simulink model "track_generator"  (R2022b)
settings: Solver=VariableStepAuto  StartTime=0.0  StopTime=120  RelTol=1e-3
values from neighbouring files (symbols this model uses):
  v_ref = 5    [trajectory_test.m]
  wp = wpt(L,vx_ref)    [trajectory_test_2.m]    (also in vehicle_lateral_control_LMIs_3states.m = wpt(L,vx_track); vehicle_lateral_control_LMIs_3states_auto.m = wpt(L,vx_track))
settings Model: Creator=phatdo  LastModifiedBy=phatdo
settings DataIOCC: ReturnWorkspaceOutputs=off

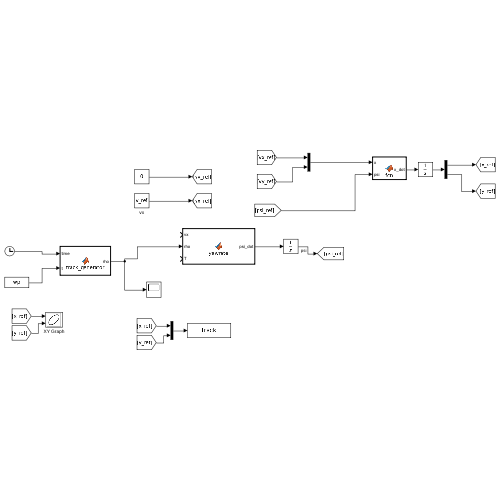
[thumbnail: Simulink's stored preview of the top-level diagram]
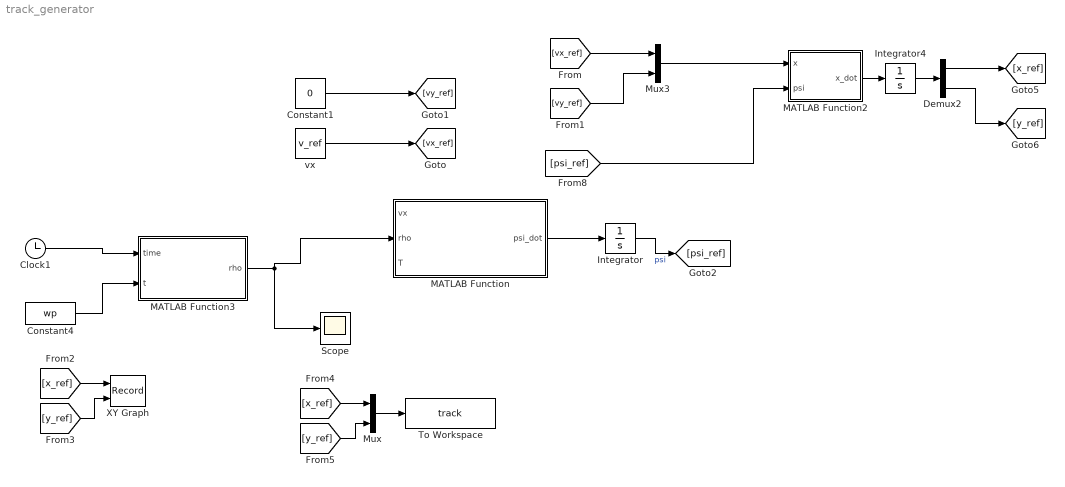
== system track_generator ==
  Clock1 : Clock
  Constant1 : Constant  Value=0
  Constant4 : Constant  Value=wp
  Demux2 : Demux  Outputs=2
  Integrator : Integrator
  Integrator4 : Integrator
  MATLAB Function : MATLAB Function  TreatAsAtomicUnit=on
  MATLAB Function2 : MATLAB Function  TreatAsAtomicUnit=on
  MATLAB Function3 : MATLAB Function  TreatAsAtomicUnit=on
  Mux : Mux  Inputs=2
  Mux3 : Mux  Inputs=2
  Scope : Scope
  To Workspace : ToWorkspace  VariableName=track  SaveFormat=Timeseries  SampleTime=-1
  XY Graph : Record  FileSettingsInternal="{\"entries\":[{\"content\":{\"excelSettings\":{\"content\":{},\"type\":\"Streamout.ExcelSettings\"}},\"type\":\"Streamout.FileSettingStorage\",\"uuid\":\"d2604bc3-c04d-4145-9e1e-7ef3e8a79466\"}],\"packageUris\":[\"http://schema.mathworks.com/mf0/streamout_blocks/R2020a\"],\"version\":\"1.0\"}"  Layout=[1 1]  SignalsInternal="{\"entries\":[{\"content\":{\"signals\":[{\"content\":{\"blockPath\":[\"track_generator/XY Graph\"],\"channel\":[],\"dimensions\":[1],\"domain\":\"track_generator/XY Graph\",\"lineColor\":\"#a2142f\",\"plots\":[1],\"port\":1,\"sid\":[\"\"],\"signalID\":2416,\"signalName\":\"From2\"},\"type\":\"RecordBlkView.Signal\",\"uuid\":\"71c5e8a0-0e4a-447b-b961-254ba126680b\"},{\"content\":{\"blockPath\":[\"track_generator/XY Graph\"],\"channel\":[],\"dimensions\":[1],\"domain\":\"track_generator/XY Graph\",\"lineColor\":\"#139fff\",\"plots\":[1],\"port\":2,\"sid\":[\"\"],\"signalID\":2420,\"signalName\":\"From3\"},\"type\":\"RecordBlkView.Signal\",\"uuid\":\"bf7e20e6-4e60-4046-b22e-00f2cb18ee01\"}]},\"type\":\"RecordBlkView.InputSignals\",\"uuid\":\"e25cf098-9fb5-4c63-b23a-ebd85c079d21\"}],\"packageUris\":[\"http://schema.mathworks.com/mf0/streamout_blocks/R2020a\"],\"version\":\"1.0\"}"  VisualizationBindings="{\"xyplotplugin\":{\"info\":[{\"series\":[{\"bindingParametersList\":[{\"parameter\":\"X-Axis\",\"signalID\":2416,\"signalName\":\"From2\"},{\"parameter\":\"Y-Axis\",\"signalID\":2420,\"signalName\":\"From3\"}],\"seriesID\":40993}],\"subplotID\":1}]}}"  CompatibilityTag=XY
  vx : Constant  Value=v_ref
  wires:
  MATLAB Function/1(psi_dot) -> Integrator/1
  vx/1 -> [vx_ref]
  Integrator/1 -> [psi_ref]  "psi"
  [vy_ref] -> Mux3/2
  Integrator4/1 -> Demux2/1
  MATLAB Function2/1(x_dot) -> Integrator4/1
  Demux2/1 -> [x_ref]
  Demux2/2 -> [y_ref]
  [psi_ref] -> MATLAB Function2/2(psi)
  [vx_ref] -> Mux3/1
  Mux3/1 -> MATLAB Function2/1(x)
  Constant1/1 -> [vy_ref]
  [y_ref] -> XY Graph/2
  [x_ref] -> XY Graph/1
  Clock1/1 -> MATLAB Function3/1(time)
  Constant4/1 -> MATLAB Function3/2(t)
  MATLAB Function3/1(rho) -> MATLAB Function/2(rho), Scope/1
  Mux/1 -> To Workspace/1
  [x_ref] -> Mux/1
  [y_ref] -> Mux/2

== matlab function track_generator/MATLAB Function3 ==
  data: time input; t input; rho output
function rho = track_generator(time,t)


rho = 0;
clothoide_const = 2600;
R = 0;
vx = 5;

if time >= t(1) && time < t(2) 
    rho = 0;% go straight
elseif time >= t(2) && time < t(3)
    rho = -vx*(time - t(2))/clothoide_const; % clothoide cornering
elseif time >= t(3) && time < t(4)
%     rho = -1/R; % circle cornering
      rho = -vx*(t(3) - t(2))/clothoide_const; % circle cornering
elseif time >= t(4) && time < t(5)
    rho = 0;% go straight
elseif time >= t(5) && time < t(6)
    rho = -vx*(time - t(5))/clothoide_const; % clothoide cornering
elseif time >= t(6) && time < t(7)
    rho = -vx*(t(6) - t(5))/clothoide_const; % circle cornering
elseif time >= t(7) && time < t(8)
    rho = 0;
elseif time >= t(8) && time < t(9)
    rho = vx*(time - t(8))/clothoide_const; % clothoide cornering
elseif time >= t(9) && time < t(10)
    rho = vx*(t(9) - t(8))/clothoide_const; % circle cornering
else
    rho = 0;
end


end

== matlab function track_generator/MATLAB Function ==
  data: vx input; psi_dot output; rho input; T input
function psi_dot = yawrate(vx, rho, T)
    psi_dot = rho*vx; % Yaw rate
end

== matlab function track_generator/MATLAB Function2 ==
  data: x input; x_dot output; psi input
function x_dot = fcn(x, psi)

% x = [vx, vy]

x_dot = zeros(2,1);

vx = x(1);
vy = x(2);

x_dot(1) = vx*cos(psi) - vy*sin(psi);
x_dot(2) = vx*sin(psi) + vy*cos(psi);

end
